simulink model "current"  (R2021a)
settings: Solver=VariableStepAuto  StartTime=0.0  StopTime=1  RelTol=1e-3
model workspace (MAT data in the model file):
  Vdc = 30
undefined symbols (not defined in the file or in its folder): f_pwm
libraries: pid_lib x5, spsControlledVoltageSourceLib x2, spsGroundLib x2, spsPermanentMagnetSynchronousMachineLib x2, spsThreePhaseVIMeasurementLib x2, spsUniversalBridgeLib x2, spsTriangleGeneratorLib x2, spsabctodq0Lib x1, spspowerguiLib x1
settings Model: SimulationMode=accelerator  Creator=Zzx  LastModifiedBy=Zzx
settings SolverCC: ZeroCrossAlgorithm=Adaptive
settings DebuggingCC: IgnoredZcDiagnostic=none

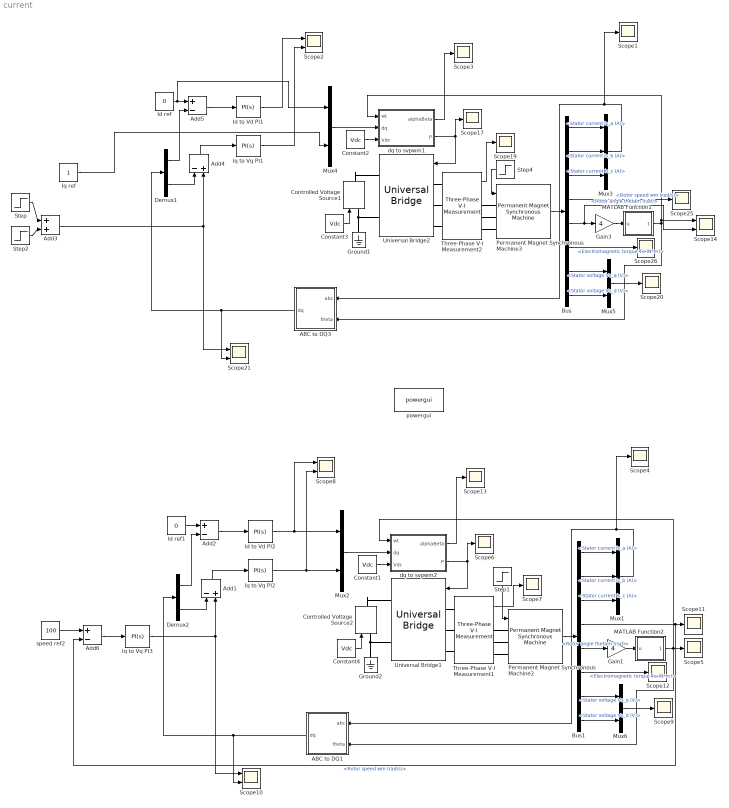
== system current ==
  ABC to DQ1 : Subsystem
  ABC to DQ3 : Subsystem
  Add1 : Sum  Inputs=-+
  Add2 : Sum  Inputs=+-
  Add3 : Sum
  Add4 : Sum  Inputs=-+
  Add5 : Sum  Inputs=+-
  Add6 : Sum  Inputs=+-
  Bus : BusSelector  OutputSignals=Stator current is_a (A),Stator current is_b (A),Stator current is_c (A),Rotor speed wm (rad/s),Rotor angle thetam (rad),Electromagnetic torque Te (N*m),Stator voltage Vs_q (V),Stator voltage Vs_d (V)
  Bus1 : BusSelector  OutputSignals=Stator current is_a (A),Stator current is_b (A),Stator current is_c (A),Rotor speed wm (rad/s),Rotor angle thetam (rad),Electromagnetic torque Te (N*m),Stator voltage Vs_q (V),Stator voltage Vs_d (V)
  Constant{1..4} (4 alike) : Constant  Value=Vdc
  Controlled Voltage Source1 : spsControlledVoltageSourceLib/Controlled Voltage Source  Initialize=on  Source_Type=DC  Amplitude=0  Phase=0  Frequency=0  Measurements=Voltage
  Controlled Voltage Source2 : spsControlledVoltageSourceLib/Controlled Voltage Source  Initialize=on  Source_Type=DC  Amplitude=0  Phase=0  Frequency=0  Measurements=Voltage
  Demux1 : Demux  Outputs=2
  Demux2 : Demux  Outputs=2
  Gain1 : Gain  Gain=4
  Gain3 : Gain  Gain=4
  Ground1 : spsGroundLib/Ground  LConnTagsString=a
  Ground2 : spsGroundLib/Ground  LConnTagsString=a
  Id ref : Constant  Value=0
  Id ref1 : Constant  Value=0
  Id to Vd PI1 : pid_lib/PID Controller  Controller=PI  Form=Parallel  TimeDomain=Continuous-time  UseExternalTs=off  SampleTime=1/f_pwm  IntegratorMethod=Forward Euler  FilterMethod=Forward Euler  ControllerParametersSource=internal  P=10  I=0  D=0  UseFilter=on  N=100  TunerSelectOption=Transfer Function Based (PID Tuner App)  InitialConditionSource=internal  InitialConditionForIntegrator=0  InitialConditionForFilter=0  DifferentiatorICPrevScaledInput=0  ExternalReset=none  TrackingMode=off  Kt=1  LimitOutput=off  SatLimitsSource=internal  UpperSaturationLimit=inf  LowerSaturationLimit=-inf  LinearizeAsGain=on  AntiWindupMode=none  Kb=1  POutMin=[]  POutMax=[]  IOutMin=[]  IOutMax=[]  DOutMin=[]  DOutMax=[]  NOutMin=[]  NOutMax=[]  SumOutMin=[]  SumOutMax=[]  SaturationOutMin=[]  SaturationOutMax=[]  PParamMin=[]  PParamMax=[]  IParamMin=[]  IParamMax=[]  DParamMin=[]  DParamMax=[]  NParamMin=[]  NParamMax=[]  KbParamMin=[]  KbParamMax=[]  KtParamMin=[]  KtParamMax=[]  KbOutMin=[]  KbOutMax=[]  KtOutMin=[]  KtOutMax=[]  IntegratorOutMin=[]  IntegratorOutMax=[]  FilterOutMin=[]  FilterOutMax=[]  SumI1OutMin=[]  SumI1OutMax=[]  SumI2OutMin=[]  SumI2OutMax=[]  SumI3OutMin=[]  SumI3OutMax=[]  SumI4OutMin=[]  SumI4OutMax=[]  SumDOutMin=[]  SumDOutMax=[]  DifferentiatorOutMin=[]  DifferentiatorOutMax=[]  FilterDiffOutCoefMin=[]  FilterDiffOutCoefMax=[]  ReciprocalOutMin=[]  ReciprocalOutMax=[]  SumDenOutMin=[]  SumDenOutMax=[]  SumNumOutMin=[]  SumNumOutMax=[]  DivideOutMin=[]  DivideOutMax=[]  UdiffTsProdOutMin=[]  UdiffTsProdOutMax=[]  NTsProdOutMin=[]  NTsProdOutMax=[]  UintegralTsProdOutMin=[]  UintegralTsProdOutMax=[]  UngainTsProdOutMin=[]  UngainTsProdOutMax=[]  IntegratorContinuousStateAttributes=''  IntegratorStateMustResolveToSignalObject=off  IntegratorRTWStateStorageClass=Auto  FilterContinuousStateAttributes=''  FilterStateMustResolveToSignalObject=off  FilterRTWStateStorageClass=Auto  ParallelPVariant=InternalParameters  IdealPVariant=Disabled  IVariant=InternalParameters  DVariant=Disabled  IntegratorVariant=Continuous  SatVariant=Disabled  AWVariant=Passthrough  PCopyVariant=Disabled  TRVariant=Disabled  FdbkBlocksVariant=Forward  IdealPFdbkVariant=Disabled  SatFdbkVariant=Disabled  DerivativeFilterVariant=Disabled  NVariant=Disabled  NCopyVariant=Disabled_SignalSpec  FilterICVariant=Disabled  IntegratorICVariant=InternalICs  ExternalResetVariant=Disabled  TRSumVariant=Passthrough  SumFdbkVariant=Disabled  SumVariant=Sum_PI  TsampFilterVariant=InternalTs  TsampNgainVariant=Passthrough  TsampIntegralVariant=Passthrough  ExternalSaturationOutDataTypeStr=Inherit: Same as second input
  Id to Vd PI2 : pid_lib/PID Controller  Controller=PI  Form=Parallel  TimeDomain=Continuous-time  UseExternalTs=off  SampleTime=1/f_pwm  IntegratorMethod=Forward Euler  FilterMethod=Forward Euler  ControllerParametersSource=internal  P=10  I=0  D=0  UseFilter=on  N=100  TunerSelectOption=Transfer Function Based (PID Tuner App)  InitialConditionSource=internal  InitialConditionForIntegrator=0  InitialConditionForFilter=0  DifferentiatorICPrevScaledInput=0  ExternalReset=none  TrackingMode=off  Kt=1  LimitOutput=off  SatLimitsSource=internal  UpperSaturationLimit=inf  LowerSaturationLimit=-inf  LinearizeAsGain=on  AntiWindupMode=none  Kb=1  POutMin=[]  POutMax=[]  IOutMin=[]  IOutMax=[]  DOutMin=[]  DOutMax=[]  NOutMin=[]  NOutMax=[]  SumOutMin=[]  SumOutMax=[]  SaturationOutMin=[]  SaturationOutMax=[]  PParamMin=[]  PParamMax=[]  IParamMin=[]  IParamMax=[]  DParamMin=[]  DParamMax=[]  NParamMin=[]  NParamMax=[]  KbParamMin=[]  KbParamMax=[]  KtParamMin=[]  KtParamMax=[]  KbOutMin=[]  KbOutMax=[]  KtOutMin=[]  KtOutMax=[]  IntegratorOutMin=[]  IntegratorOutMax=[]  FilterOutMin=[]  FilterOutMax=[]  SumI1OutMin=[]  SumI1OutMax=[]  SumI2OutMin=[]  SumI2OutMax=[]  SumI3OutMin=[]  SumI3OutMax=[]  SumI4OutMin=[]  SumI4OutMax=[]  SumDOutMin=[]  SumDOutMax=[]  DifferentiatorOutMin=[]  DifferentiatorOutMax=[]  FilterDiffOutCoefMin=[]  FilterDiffOutCoefMax=[]  ReciprocalOutMin=[]  ReciprocalOutMax=[]  SumDenOutMin=[]  SumDenOutMax=[]  SumNumOutMin=[]  SumNumOutMax=[]  DivideOutMin=[]  DivideOutMax=[]  UdiffTsProdOutMin=[]  UdiffTsProdOutMax=[]  NTsProdOutMin=[]  NTsProdOutMax=[]  UintegralTsProdOutMin=[]  UintegralTsProdOutMax=[]  UngainTsProdOutMin=[]  UngainTsProdOutMax=[]  IntegratorContinuousStateAttributes=''  IntegratorStateMustResolveToSignalObject=off  IntegratorRTWStateStorageClass=Auto  FilterContinuousStateAttributes=''  FilterStateMustResolveToSignalObject=off  FilterRTWStateStorageClass=Auto  ParallelPVariant=InternalParameters  IdealPVariant=Disabled  IVariant=InternalParameters  DVariant=Disabled  IntegratorVariant=Continuous  SatVariant=Disabled  AWVariant=Passthrough  PCopyVariant=Disabled  TRVariant=Disabled  FdbkBlocksVariant=Forward  IdealPFdbkVariant=Disabled  SatFdbkVariant=Disabled  DerivativeFilterVariant=Disabled  NVariant=Disabled  NCopyVariant=Disabled_SignalSpec  FilterICVariant=Disabled  IntegratorICVariant=InternalICs  ExternalResetVariant=Disabled  TRSumVariant=Passthrough  SumFdbkVariant=Disabled  SumVariant=Sum_PI  TsampFilterVariant=InternalTs  TsampNgainVariant=Passthrough  TsampIntegralVariant=Passthrough  ExternalSaturationOutDataTypeStr=Inherit: Same as second input
  Iq ref : Constant
  Iq to Vq PI1 : pid_lib/PID Controller  Controller=PI  Form=Parallel  TimeDomain=Continuous-time  UseExternalTs=off  SampleTime=1/f_pwm  IntegratorMethod=Forward Euler  FilterMethod=Forward Euler  ControllerParametersSource=internal  P=10  I=0  D=0  UseFilter=on  N=100  TunerSelectOption=Transfer Function Based (PID Tuner App)  InitialConditionSource=internal  InitialConditionForIntegrator=0  InitialConditionForFilter=0  DifferentiatorICPrevScaledInput=0  ExternalReset=none  TrackingMode=off  Kt=1  LimitOutput=off  SatLimitsSource=internal  UpperSaturationLimit=inf  LowerSaturationLimit=-inf  LinearizeAsGain=on  AntiWindupMode=none  Kb=1  POutMin=[]  POutMax=[]  IOutMin=[]  IOutMax=[]  DOutMin=[]  DOutMax=[]  NOutMin=[]  NOutMax=[]  SumOutMin=[]  SumOutMax=[]  SaturationOutMin=[]  SaturationOutMax=[]  PParamMin=[]  PParamMax=[]  IParamMin=[]  IParamMax=[]  DParamMin=[]  DParamMax=[]  NParamMin=[]  NParamMax=[]  KbParamMin=[]  KbParamMax=[]  KtParamMin=[]  KtParamMax=[]  KbOutMin=[]  KbOutMax=[]  KtOutMin=[]  KtOutMax=[]  IntegratorOutMin=[]  IntegratorOutMax=[]  FilterOutMin=[]  FilterOutMax=[]  SumI1OutMin=[]  SumI1OutMax=[]  SumI2OutMin=[]  SumI2OutMax=[]  SumI3OutMin=[]  SumI3OutMax=[]  SumI4OutMin=[]  SumI4OutMax=[]  SumDOutMin=[]  SumDOutMax=[]  DifferentiatorOutMin=[]  DifferentiatorOutMax=[]  FilterDiffOutCoefMin=[]  FilterDiffOutCoefMax=[]  ReciprocalOutMin=[]  ReciprocalOutMax=[]  SumDenOutMin=[]  SumDenOutMax=[]  SumNumOutMin=[]  SumNumOutMax=[]  DivideOutMin=[]  DivideOutMax=[]  UdiffTsProdOutMin=[]  UdiffTsProdOutMax=[]  NTsProdOutMin=[]  NTsProdOutMax=[]  UintegralTsProdOutMin=[]  UintegralTsProdOutMax=[]  UngainTsProdOutMin=[]  UngainTsProdOutMax=[]  IntegratorContinuousStateAttributes=''  IntegratorStateMustResolveToSignalObject=off  IntegratorRTWStateStorageClass=Auto  FilterContinuousStateAttributes=''  FilterStateMustResolveToSignalObject=off  FilterRTWStateStorageClass=Auto  ParallelPVariant=InternalParameters  IdealPVariant=Disabled  IVariant=InternalParameters  DVariant=Disabled  IntegratorVariant=Continuous  SatVariant=Disabled  AWVariant=Passthrough  PCopyVariant=Disabled  TRVariant=Disabled  FdbkBlocksVariant=Forward  IdealPFdbkVariant=Disabled  SatFdbkVariant=Disabled  DerivativeFilterVariant=Disabled  NVariant=Disabled  NCopyVariant=Disabled_SignalSpec  FilterICVariant=Disabled  IntegratorICVariant=InternalICs  ExternalResetVariant=Disabled  TRSumVariant=Passthrough  SumFdbkVariant=Disabled  SumVariant=Sum_PI  TsampFilterVariant=InternalTs  TsampNgainVariant=Passthrough  TsampIntegralVariant=Passthrough  ExternalSaturationOutDataTypeStr=Inherit: Same as second input
  Iq to Vq PI2 : pid_lib/PID Controller  Controller=PI  Form=Parallel  TimeDomain=Continuous-time  UseExternalTs=off  SampleTime=1/f_pwm  IntegratorMethod=Forward Euler  FilterMethod=Forward Euler  ControllerParametersSource=internal  P=10  I=0  D=0  UseFilter=on  N=100  TunerSelectOption=Transfer Function Based (PID Tuner App)  InitialConditionSource=internal  InitialConditionForIntegrator=0  InitialConditionForFilter=0  DifferentiatorICPrevScaledInput=0  ExternalReset=none  TrackingMode=off  Kt=1  LimitOutput=off  SatLimitsSource=internal  UpperSaturationLimit=inf  LowerSaturationLimit=-inf  LinearizeAsGain=on  AntiWindupMode=none  Kb=1  POutMin=[]  POutMax=[]  IOutMin=[]  IOutMax=[]  DOutMin=[]  DOutMax=[]  NOutMin=[]  NOutMax=[]  SumOutMin=[]  SumOutMax=[]  SaturationOutMin=[]  SaturationOutMax=[]  PParamMin=[]  PParamMax=[]  IParamMin=[]  IParamMax=[]  DParamMin=[]  DParamMax=[]  NParamMin=[]  NParamMax=[]  KbParamMin=[]  KbParamMax=[]  KtParamMin=[]  KtParamMax=[]  KbOutMin=[]  KbOutMax=[]  KtOutMin=[]  KtOutMax=[]  IntegratorOutMin=[]  IntegratorOutMax=[]  FilterOutMin=[]  FilterOutMax=[]  SumI1OutMin=[]  SumI1OutMax=[]  SumI2OutMin=[]  SumI2OutMax=[]  SumI3OutMin=[]  SumI3OutMax=[]  SumI4OutMin=[]  SumI4OutMax=[]  SumDOutMin=[]  SumDOutMax=[]  DifferentiatorOutMin=[]  DifferentiatorOutMax=[]  FilterDiffOutCoefMin=[]  FilterDiffOutCoefMax=[]  ReciprocalOutMin=[]  ReciprocalOutMax=[]  SumDenOutMin=[]  SumDenOutMax=[]  SumNumOutMin=[]  SumNumOutMax=[]  DivideOutMin=[]  DivideOutMax=[]  UdiffTsProdOutMin=[]  UdiffTsProdOutMax=[]  NTsProdOutMin=[]  NTsProdOutMax=[]  UintegralTsProdOutMin=[]  UintegralTsProdOutMax=[]  UngainTsProdOutMin=[]  UngainTsProdOutMax=[]  IntegratorContinuousStateAttributes=''  IntegratorStateMustResolveToSignalObject=off  IntegratorRTWStateStorageClass=Auto  FilterContinuousStateAttributes=''  FilterStateMustResolveToSignalObject=off  FilterRTWStateStorageClass=Auto  ParallelPVariant=InternalParameters  IdealPVariant=Disabled  IVariant=InternalParameters  DVariant=Disabled  IntegratorVariant=Continuous  SatVariant=Disabled  AWVariant=Passthrough  PCopyVariant=Disabled  TRVariant=Disabled  FdbkBlocksVariant=Forward  IdealPFdbkVariant=Disabled  SatFdbkVariant=Disabled  DerivativeFilterVariant=Disabled  NVariant=Disabled  NCopyVariant=Disabled_SignalSpec  FilterICVariant=Disabled  IntegratorICVariant=InternalICs  ExternalResetVariant=Disabled  TRSumVariant=Passthrough  SumFdbkVariant=Disabled  SumVariant=Sum_PI  TsampFilterVariant=InternalTs  TsampNgainVariant=Passthrough  TsampIntegralVariant=Passthrough  ExternalSaturationOutDataTypeStr=Inherit: Same as second input
  Iq to Vq PI3 : pid_lib/PID Controller  Controller=PI  Form=Parallel  TimeDomain=Continuous-time  UseExternalTs=off  SampleTime=1/f_pwm  IntegratorMethod=Forward Euler  FilterMethod=Forward Euler  ControllerParametersSource=internal  P=10  I=0  D=0  UseFilter=on  N=100  TunerSelectOption=Transfer Function Based (PID Tuner App)  InitialConditionSource=internal  InitialConditionForIntegrator=0  InitialConditionForFilter=0  DifferentiatorICPrevScaledInput=0  ExternalReset=none  TrackingMode=off  Kt=1  LimitOutput=off  SatLimitsSource=internal  UpperSaturationLimit=inf  LowerSaturationLimit=-inf  LinearizeAsGain=on  AntiWindupMode=none  Kb=1  POutMin=[]  POutMax=[]  IOutMin=[]  IOutMax=[]  DOutMin=[]  DOutMax=[]  NOutMin=[]  NOutMax=[]  SumOutMin=[]  SumOutMax=[]  SaturationOutMin=[]  SaturationOutMax=[]  PParamMin=[]  PParamMax=[]  IParamMin=[]  IParamMax=[]  DParamMin=[]  DParamMax=[]  NParamMin=[]  NParamMax=[]  KbParamMin=[]  KbParamMax=[]  KtParamMin=[]  KtParamMax=[]  KbOutMin=[]  KbOutMax=[]  KtOutMin=[]  KtOutMax=[]  IntegratorOutMin=[]  IntegratorOutMax=[]  FilterOutMin=[]  FilterOutMax=[]  SumI1OutMin=[]  SumI1OutMax=[]  SumI2OutMin=[]  SumI2OutMax=[]  SumI3OutMin=[]  SumI3OutMax=[]  SumI4OutMin=[]  SumI4OutMax=[]  SumDOutMin=[]  SumDOutMax=[]  DifferentiatorOutMin=[]  DifferentiatorOutMax=[]  FilterDiffOutCoefMin=[]  FilterDiffOutCoefMax=[]  ReciprocalOutMin=[]  ReciprocalOutMax=[]  SumDenOutMin=[]  SumDenOutMax=[]  SumNumOutMin=[]  SumNumOutMax=[]  DivideOutMin=[]  DivideOutMax=[]  UdiffTsProdOutMin=[]  UdiffTsProdOutMax=[]  NTsProdOutMin=[]  NTsProdOutMax=[]  UintegralTsProdOutMin=[]  UintegralTsProdOutMax=[]  UngainTsProdOutMin=[]  UngainTsProdOutMax=[]  IntegratorContinuousStateAttributes=''  IntegratorStateMustResolveToSignalObject=off  IntegratorRTWStateStorageClass=Auto  FilterContinuousStateAttributes=''  FilterStateMustResolveToSignalObject=off  FilterRTWStateStorageClass=Auto  ParallelPVariant=InternalParameters  IdealPVariant=Disabled  IVariant=InternalParameters  DVariant=Disabled  IntegratorVariant=Continuous  SatVariant=Disabled  AWVariant=Passthrough  PCopyVariant=Disabled  TRVariant=Disabled  FdbkBlocksVariant=Forward  IdealPFdbkVariant=Disabled  SatFdbkVariant=Disabled  DerivativeFilterVariant=Disabled  NVariant=Disabled  NCopyVariant=Disabled_SignalSpec  FilterICVariant=Disabled  IntegratorICVariant=InternalICs  ExternalResetVariant=Disabled  TRSumVariant=Passthrough  SumFdbkVariant=Disabled  SumVariant=Sum_PI  TsampFilterVariant=InternalTs  TsampNgainVariant=Passthrough  TsampIntegralVariant=Passthrough  ExternalSaturationOutDataTypeStr=Inherit: Same as second input
  MATLAB Function1 : MATLAB Function  TreatAsAtomicUnit=on
  MATLAB Function2 : MATLAB Function  TreatAsAtomicUnit=on
  Mux1 : Mux  Inputs=3
  Mux{2,4..6} (4 alike) : Mux  Inputs=2
  Mux3 : Mux  Inputs=3
  Permanent Magnet Synchronous Machine2 : spsPermanentMagnetSynchronousMachineLib/Permanent Magnet Synchronous Machine  NbPhases=3  FluxDistribution=Sinusoidal  RotorType=Round  MechanicalLoad=Torque Tm  PresetModel=No  ShowDetailedParameters=on  MeasurementBus=off  Resistance=0.89  Inductance=8.5e-3  dqInductances=[8.5e-3,8.5e-3]  La=0.00062  MachineConstant=Voltage Constant (V_peak L-L / krpm)  Flux=0.0056925  VoltageCst=4.13  TorqueCst=0.034155  Flat=120  Mechanical=[ 0.8e-3, 0 4]  PolePairs=4  InitialConditions=[0,0, 0,0]  InitialConditions5ph=[0 0 0 0 0 0]  RefAngle=Aligned with phase A axis (original Park)  IterativeDiscreteModel=Trapezoidal non iterative  TsBlock=-1  TsPowergui=0
  Permanent Magnet Synchronous Machine3 : spsPermanentMagnetSynchronousMachineLib/Permanent Magnet Synchronous Machine  NbPhases=3  FluxDistribution=Sinusoidal  RotorType=Round  MechanicalLoad=Torque Tm  PresetModel=No  ShowDetailedParameters=on  MeasurementBus=off  Resistance=0.89  Inductance=8.5e-3  dqInductances=[8.5e-3,8.5e-3]  La=0.00062  MachineConstant=Voltage Constant (V_peak L-L / krpm)  Flux=0.0056925  VoltageCst=4.13  TorqueCst=0.034155  Flat=120  Mechanical=[ 0.8e-3, 0 4]  PolePairs=4  InitialConditions=[0,0, 0,0]  InitialConditions5ph=[0 0 0 0 0 0]  RefAngle=Aligned with phase A axis (original Park)  IterativeDiscreteModel=Trapezoidal non iterative  TsBlock=-1  TsPowergui=0
  Scope{1,3..7,9,11..13,17,19..20,25..26} (15 alike) : Scope
  Scope{2,8,10,14,21} (5 alike) : Scope  NumInputPorts=2
  Step : Step  Time=0.25  Before=0.5  After=2  SampleTime=0
  Step1 : Step  Time=0.5  After=0  SampleTime=0
  Step2 : Step  Time=0.75  After=-1  SampleTime=0
  Step4 : Step  Time=0.5  After=0  SampleTime=0
  Three-Phase V-I Measurement1 : spsThreePhaseVIMeasurementLib/Three-Phase V-I Measurement  VoltageMeasurement=phase-to-ground  SetLabelV=off  LabelV=Vabc  Vpu=off  VpuLL=off  CurrentMeasurement=yes  SetLabelI=off  LabelI=Iabc  Ipu=off  Pbase=100e6  Vbase=500e3  OutputType=Complex  PhasorSimulation=off  PSBequivalent=0
  Three-Phase V-I Measurement2 : spsThreePhaseVIMeasurementLib/Three-Phase V-I Measurement  VoltageMeasurement=phase-to-ground  SetLabelV=off  LabelV=Vabc  Vpu=off  VpuLL=off  CurrentMeasurement=yes  SetLabelI=off  LabelI=Iabc  Ipu=off  Pbase=100e6  Vbase=500e3  OutputType=Complex  PhasorSimulation=off  PSBequivalent=0
  Universal Bridge1 : spsUniversalBridgeLib/Universal Bridge  Arms=3  SnubberResistance=1e5  SnubberCapacitance=inf  Device=IGBT / Diodes  Ron=1e-3  Lon=0  ForwardVoltages="[  0  0  ]"  ForwardVoltage=0  GTOparameters=[ 10e-6 , 20e-6 ]  IGBTparameters=[ 1e-6 , 2e-6 ]  Measurements=None  Measurements_2=None  converterType=Rectifier
  Universal Bridge2 : spsUniversalBridgeLib/Universal Bridge  Arms=3  SnubberResistance=1e5  SnubberCapacitance=inf  Device=IGBT / Diodes  Ron=1e-3  Lon=0  ForwardVoltages="[  0  0  ]"  ForwardVoltage=0  GTOparameters=[ 10e-6 , 20e-6 ]  IGBTparameters=[ 1e-6 , 2e-6 ]  Measurements=None  Measurements_2=None  converterType=Rectifier
  dq to svpwm1 : Subsystem
  dq to svpwm2 : Subsystem
  powergui : spspowerguiLib/powergui  Priority=1  SimulationMode=Continuous  SampleTime=50e-6  frequency=60  Iterations=50  frequencyindice=0  Pbase=100e6  ErrMax=1e-4  UnitsV=kV  UnitsW=MW  buscounter=0  FunctionMessages=off  echomessages=off  EnableUseOfTLC=off  CurrentSourceSwitches=off  DisableSnubberDevices=off  DisableRonSwitches=off  DisableVfSwitches=off  DisplayEquations=off  AutomaticDiscreteSolvers=off  SolverType=Tustin/Backward Euler (TBE)  Interpol=off  ExternalGateDelay=off  methode=off  Ts=100  x0status=blocks  SPID=on  SwTol=0  HookPort=off  NonlinearTolerance=1e-4  nMaxIteration=100  ContinueOnMaxIteration=off  RestoreLinks=warning  ResistiveCurrentMeasurement=off  Frange=[0:2:500]  Ylog=off  Xlog=on  ShowGrid=off  save=off  variable=ZData  structure=0  ZoomFFT=off  StartTime=0.0  cycles=1  DisplayStyle=1  fundamental=60  FreqAxis=off  MaxFrequency=1000  frequencyindicesteady=1  RmsSteady=1  display=off
  speed ref2 : Constant  Value=100
  wires:
  Three-Phase V-I Measurement2/1 -> Scope19/1
  Id to Vd PI1/1 -> Scope2/1
  Iq to Vq PI1/1 -> Scope2/2
  Step4/1 -> Permanent Magnet Synchronous Machine3/1
  Bus/7 -> Mux5/1  "<Stator voltage Vs_q (V)>"
  Bus/2 -> Mux3/2  "<Stator current is_b (A)>"
  Bus/5 -> Scope14/2, Gain3/1  "<Rotor angle thetam (rad)>"
  Bus/6 -> Scope26/1  "<Electromagnetic torque Te (N*m)>"
  Mux4/1 -> dq to svpwm1/2(dq)
  ABC to DQ3/1(dq) -> Scope21/2, Demux1/1
  Constant2/1 -> dq to svpwm1/3(Vdc)
  Bus/8 -> Mux5/2  "<Stator voltage Vs_d (V)>"
  Mux3/1 -> ABC to DQ3/1(abc), Scope1/1
  Gain3/1 -> MATLAB Function1/1(u)
  Bus/1 -> Mux3/1  "<Stator current is_a (A)>"
  Mux5/1 -> Scope20/1
  Add4/1 -> Iq to Vq PI1/1
  Bus/4 -> Scope25/1  "<Rotor speed wm (rad/s)>"
  Bus/3 -> Mux3/3  "<Stator current is_c (A)>"
  Demux1/2 -> Add4/1
  Id ref/1 -> Mux4/1, Add5/1
  MATLAB Function1/1(theta) -> Scope14/1, dq to svpwm1/1(wt), ABC to DQ3/2(theta)
  Add5/1 -> Id to Vd PI1/1
  Demux1/1 -> Add5/2
  Constant3/1 -> Controlled Voltage Source1/1
  dq to svpwm1/2(P) -> Scope17/1, Universal Bridge2/1
  Permanent Magnet Synchronous Machine3/1 -> Bus/1
  dq to svpwm1/1(alphaBeta) -> Scope3/1
  Add3/1 -> Scope21/1, Add4/2
  Step/1 -> Add3/1
  Step2/1 -> Add3/2
  Step1/1 -> Permanent Magnet Synchronous Machine2/1
  Permanent Magnet Synchronous Machine2/1 -> Bus1/1
  dq to svpwm2/2(P) -> Scope6/1, Universal Bridge1/1
  Demux2/1 -> Add2/2
  Id ref1/1 -> Add2/1
  Demux2/2 -> Add1/1
  Gain1/1 -> MATLAB Function2/1(u)
  Mux6/1 -> Scope9/1
  Bus1/3 -> Mux1/3  "<Stator current is_c (A)>"
  MATLAB Function2/1(theta) -> dq to svpwm2/1(wt), ABC to DQ1/2(theta), Scope5/1
  Bus1/1 -> Mux1/1  "<Stator current is_a (A)>"
  Bus1/8 -> Mux6/2  "<Stator voltage Vs_d (V)>"
  Bus1/5 -> Gain1/1  "<Rotor angle thetam (rad)>"
  Constant1/1 -> dq to svpwm2/3(Vdc)
  Add1/1 -> Iq to Vq PI2/1
  Constant4/1 -> Controlled Voltage Source2/1
  ABC to DQ1/1(dq) -> Scope10/2, Demux2/1
  Mux2/1 -> dq to svpwm2/2(dq)
  Bus1/6 -> Scope12/1  "<Electromagnetic torque Te (N*m)>"
  Three-Phase V-I Measurement1/1 -> Scope7/1
  Id to Vd PI2/1 -> Mux2/1, Scope8/1
  Iq to Vq PI2/1 -> Mux2/2, Scope8/2
  Bus1/2 -> Mux1/2  "<Stator current is_b (A)>"
  Mux1/1 -> ABC to DQ1/1(abc), Scope4/1
  Bus1/7 -> Mux6/1  "<Stator voltage Vs_q (V)>"
  dq to svpwm2/1(alphaBeta) -> Scope13/1
  Add2/1 -> Id to Vd PI2/1
  Bus1/4 -> Add6/2, Scope11/1  "<Rotor speed wm (rad/s)>"
  Iq to Vq PI3/1 -> Add1/2, Scope10/1
  speed ref2/1 -> Add6/1
  Add6/1 -> Iq to Vq PI3/1
  Iq ref/1 -> Mux4/2
  connections:
  Controlled Voltage Source1/LConn1 -- Ground1/LConn1 -- Universal Bridge2/RConn2
  Three-Phase V-I Measurement2/LConn1 -- Universal Bridge2/LConn1
  Permanent Magnet Synchronous Machine3/LConn3 -- Three-Phase V-I Measurement2/RConn3
  Three-Phase V-I Measurement2/LConn2 -- Universal Bridge2/LConn2
  Controlled Voltage Source1/RConn1 -- Universal Bridge2/RConn1
  Permanent Magnet Synchronous Machine3/LConn2 -- Three-Phase V-I Measurement2/RConn2
  Three-Phase V-I Measurement2/LConn3 -- Universal Bridge2/LConn3
  Permanent Magnet Synchronous Machine3/LConn1 -- Three-Phase V-I Measurement2/RConn1
  Controlled Voltage Source2/LConn1 -- Ground2/LConn1 -- Universal Bridge1/RConn2
  Permanent Magnet Synchronous Machine2/LConn2 -- Three-Phase V-I Measurement1/RConn2
  Permanent Magnet Synchronous Machine2/LConn1 -- Three-Phase V-I Measurement1/RConn1
  Controlled Voltage Source2/RConn1 -- Universal Bridge1/RConn1
  Three-Phase V-I Measurement1/LConn1 -- Universal Bridge1/LConn1
  Three-Phase V-I Measurement1/LConn2 -- Universal Bridge1/LConn2
  Three-Phase V-I Measurement1/LConn3 -- Universal Bridge1/LConn3
  Permanent Magnet Synchronous Machine2/LConn3 -- Three-Phase V-I Measurement1/RConn3

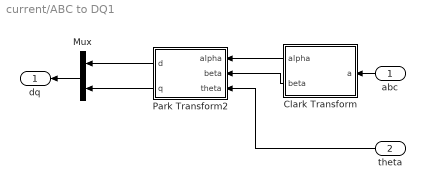
== system current/ABC to DQ1 ==
  abc : Inport
  theta : Inport  Port=2
  Clark Transform : MATLAB Function  TreatAsAtomicUnit=on
  Mux : Mux  Inputs=2
  Park Transform2 : MATLAB Function  TreatAsAtomicUnit=on
  dq : Outport
  wires:
  Clark Transform/1(alpha) -> Park Transform2/1(alpha)
  Clark Transform/2(beta) -> Park Transform2/2(beta)
  abc/1 -> Clark Transform/1(a)
  theta/1 -> Park Transform2/3(theta)
  Park Transform2/1(d) -> Mux/1
  Park Transform2/2(q) -> Mux/2
  Mux/1 -> dq/1

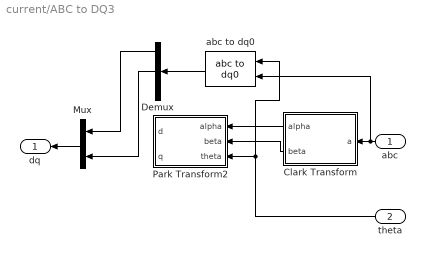
== system current/ABC to DQ3 ==
  abc : Inport
  theta : Inport  Port=2
  Clark Transform : MATLAB Function  TreatAsAtomicUnit=on
  Demux : Demux  Outputs=3
  Mux : Mux  Inputs=2
  Park Transform2 : MATLAB Function  TreatAsAtomicUnit=on
  abc to dq0 : spsabctodq0Lib/abc to dq0  Alignment=90 degrees behind phase A axis
  dq : Outport
  wires:
  Clark Transform/1(alpha) -> Park Transform2/1(alpha)
  Clark Transform/2(beta) -> Park Transform2/2(beta)
  abc/1 -> abc to dq0/1, Clark Transform/1(a)
  theta/1 -> abc to dq0/2, Park Transform2/3(theta)
  Mux/1 -> dq/1
  abc to dq0/1 -> Demux/1
  Demux/1 -> Mux/1
  Demux/2 -> Mux/2

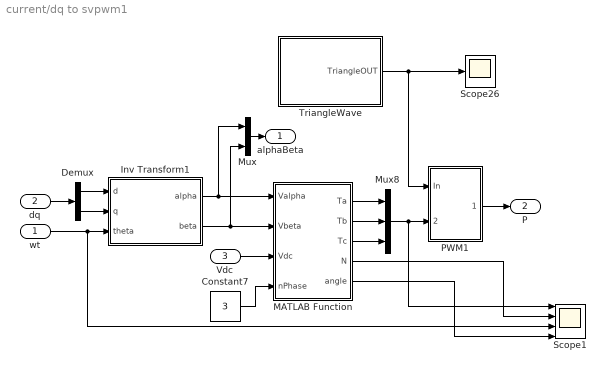
== system current/dq to svpwm1 ==
  wt : Inport
  dq : Inport  Port=2
  Vdc : Inport  Port=3
  Constant7 : Constant  Value=3
  Demux : Demux  Outputs=2
  Inv Transform1 : MATLAB Function  TreatAsAtomicUnit=on
  MATLAB Function : MATLAB Function  TreatAsAtomicUnit=on
  Mux : Mux  Inputs=2
  Mux8 : Mux  Inputs=3
  PWM1 : Subsystem
  Scope1 : Scope  NumInputPorts=4
  Scope26 : Scope
  TriangleWave : Subsystem
  alphaBeta : Outport
  P : Outport  Port=2
  wires:
  Inv Transform1/2(beta) -> MATLAB Function/2(Vbeta), Mux/2
  wt/1 -> Scope1/3, Inv Transform1/3(theta)
  dq/1 -> Demux/1
  Inv Transform1/1(alpha) -> MATLAB Function/1(Valpha), Mux/1
  MATLAB Function/1(Ta) -> Mux8/1
  MATLAB Function/3(Tc) -> Mux8/3
  MATLAB Function/2(Tb) -> Mux8/2
  Vdc/1 -> MATLAB Function/3(Vdc)
  Constant7/1 -> MATLAB Function/4(nPhase)
  PWM1/1(PWM) -> P/1
  Mux8/1 -> PWM1/2(Tcm123), Scope1/1
  Demux/1 -> Inv Transform1/1(d)
  Demux/2 -> Inv Transform1/2(q)
  Mux/1 -> alphaBeta/1
  TriangleWave/1(TriangleOUT) -> Scope26/1, PWM1/1(In)
  MATLAB Function/4(N) -> Scope1/2
  MATLAB Function/5(angle) -> Scope1/4

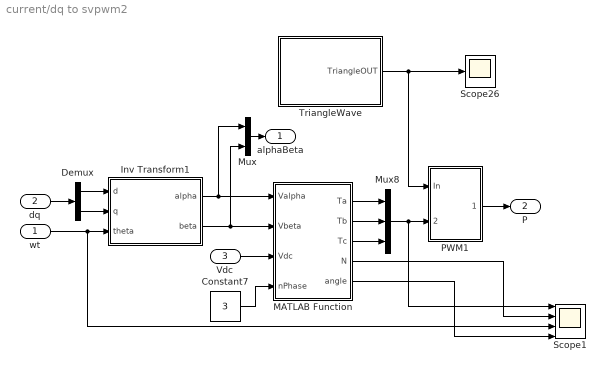
== system current/dq to svpwm2 ==
  wt : Inport
  dq : Inport  Port=2
  Vdc : Inport  Port=3
  Constant7 : Constant  Value=3
  Demux : Demux  Outputs=2
  Inv Transform1 : MATLAB Function  TreatAsAtomicUnit=on
  MATLAB Function : MATLAB Function  TreatAsAtomicUnit=on
  Mux : Mux  Inputs=2
  Mux8 : Mux  Inputs=3
  PWM1 : Subsystem
  Scope1 : Scope  NumInputPorts=4
  Scope26 : Scope
  TriangleWave : Subsystem
  alphaBeta : Outport
  P : Outport  Port=2
  wires:
  Inv Transform1/2(beta) -> MATLAB Function/2(Vbeta), Mux/2
  wt/1 -> Scope1/3, Inv Transform1/3(theta)
  dq/1 -> Demux/1
  Inv Transform1/1(alpha) -> MATLAB Function/1(Valpha), Mux/1
  MATLAB Function/1(Ta) -> Mux8/1
  MATLAB Function/3(Tc) -> Mux8/3
  MATLAB Function/2(Tb) -> Mux8/2
  Vdc/1 -> MATLAB Function/3(Vdc)
  Constant7/1 -> MATLAB Function/4(nPhase)
  PWM1/1(PWM) -> P/1
  Mux8/1 -> PWM1/2(Tcm123), Scope1/1
  Demux/1 -> Inv Transform1/1(d)
  Demux/2 -> Inv Transform1/2(q)
  Mux/1 -> alphaBeta/1
  TriangleWave/1(TriangleOUT) -> Scope26/1, PWM1/1(In)
  MATLAB Function/4(N) -> Scope1/2
  MATLAB Function/5(angle) -> Scope1/4

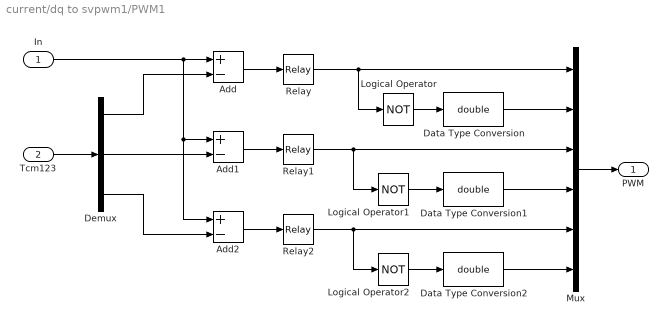
== system current/dq to svpwm1/PWM1 ==
  In : Inport
  Tcm123 : Inport  Port=2
  Add : Sum  Inputs=+-
  Add1 : Sum  Inputs=+-
  Add2 : Sum  Inputs=+-
  Data Type Conversion : DataTypeConversion  OutDataTypeStr=double
  Data Type Conversion1 : DataTypeConversion  OutDataTypeStr=double
  Data Type Conversion2 : DataTypeConversion  OutDataTypeStr=double
  Demux : Demux  Outputs=3
  Logical Operator : Logic  Operator=NOT  AllPortsSameDT=off  OutDataTypeStr=boolean
  Logical Operator1 : Logic  Operator=NOT  AllPortsSameDT=off  OutDataTypeStr=boolean
  Logical Operator2 : Logic  Operator=NOT  AllPortsSameDT=off  OutDataTypeStr=boolean
  Mux : Mux  Inputs=6
  Relay : Relay
  Relay1 : Relay
  Relay2 : Relay
  PWM : Outport
  wires:
  Demux/3 -> Add2/2
  Demux/2 -> Add1/2
  Demux/1 -> Add/2
  Relay2/1 -> Mux/5, Logical Operator2/1
  Relay1/1 -> Mux/3, Logical Operator1/1
  Relay/1 -> Logical Operator/1, Mux/1
  Mux/1 -> PWM/1
  Data Type Conversion/1 -> Mux/2
  Data Type Conversion1/1 -> Mux/4
  Data Type Conversion2/1 -> Mux/6
  Logical Operator2/1 -> Data Type Conversion2/1
  Logical Operator1/1 -> Data Type Conversion1/1
  Logical Operator/1 -> Data Type Conversion/1
  Add1/1 -> Relay1/1
  Add2/1 -> Relay2/1
  Add/1 -> Relay/1
  In/1 -> Add/1, Add2/1, Add1/1
  Tcm123/1 -> Demux/1

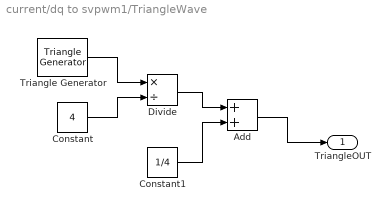
== system current/dq to svpwm1/TriangleWave ==
  Add : Sum
  Constant : Constant  Value=4
  Constant1 : Constant  Value=1/4
  Divide : Product  Inputs=*/
  Triangle Generator : spsTriangleGeneratorLib/Triangle Generator  Freq=f_pwm  Phase=0  Ts=0
  TriangleOUT : Outport
  wires:
  Add/1 -> TriangleOUT/1
  Constant/1 -> Divide/2
  Constant1/1 -> Add/2
  Divide/1 -> Add/1
  Triangle Generator/1 -> Divide/1

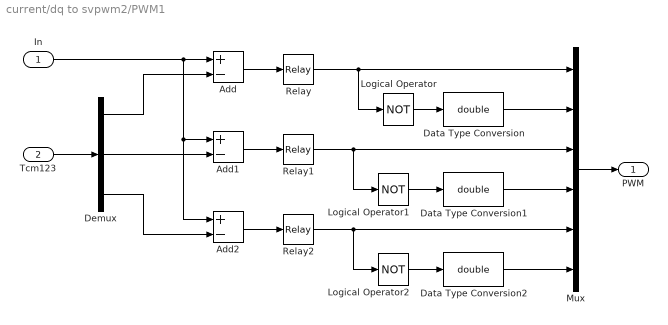
== system current/dq to svpwm2/PWM1 ==
  In : Inport
  Tcm123 : Inport  Port=2
  Add : Sum  Inputs=+-
  Add1 : Sum  Inputs=+-
  Add2 : Sum  Inputs=+-
  Data Type Conversion : DataTypeConversion  OutDataTypeStr=double
  Data Type Conversion1 : DataTypeConversion  OutDataTypeStr=double
  Data Type Conversion2 : DataTypeConversion  OutDataTypeStr=double
  Demux : Demux  Outputs=3
  Logical Operator : Logic  Operator=NOT  AllPortsSameDT=off  OutDataTypeStr=boolean
  Logical Operator1 : Logic  Operator=NOT  AllPortsSameDT=off  OutDataTypeStr=boolean
  Logical Operator2 : Logic  Operator=NOT  AllPortsSameDT=off  OutDataTypeStr=boolean
  Mux : Mux  Inputs=6
  Relay : Relay
  Relay1 : Relay
  Relay2 : Relay
  PWM : Outport
  wires:
  Demux/3 -> Add2/2
  Demux/2 -> Add1/2
  Demux/1 -> Add/2
  Relay2/1 -> Mux/5, Logical Operator2/1
  Relay1/1 -> Mux/3, Logical Operator1/1
  Relay/1 -> Logical Operator/1, Mux/1
  Mux/1 -> PWM/1
  Data Type Conversion/1 -> Mux/2
  Data Type Conversion1/1 -> Mux/4
  Data Type Conversion2/1 -> Mux/6
  Logical Operator2/1 -> Data Type Conversion2/1
  Logical Operator1/1 -> Data Type Conversion1/1
  Logical Operator/1 -> Data Type Conversion/1
  Add1/1 -> Relay1/1
  Add2/1 -> Relay2/1
  Add/1 -> Relay/1
  In/1 -> Add/1, Add2/1, Add1/1
  Tcm123/1 -> Demux/1

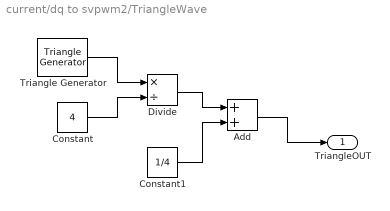
== system current/dq to svpwm2/TriangleWave ==
  Add : Sum
  Constant : Constant  Value=4
  Constant1 : Constant  Value=1/4
  Divide : Product  Inputs=*/
  Triangle Generator : spsTriangleGeneratorLib/Triangle Generator  Freq=f_pwm  Phase=0  Ts=0
  TriangleOUT : Outport
  wires:
  Add/1 -> TriangleOUT/1
  Constant/1 -> Divide/2
  Constant1/1 -> Add/2
  Divide/1 -> Add/1
  Triangle Generator/1 -> Divide/1

== matlab function current/ABC to DQ1/Clark Transform ==
  data: a input; alpha output; beta output
function [alpha,beta] = fcn(a)

alpha = a(1)-0.5*a(2)-0.5*a(3);
beta = 0.5*sqrt(3)*a(2)-0.5*sqrt(3)*a(3);

== matlab function current/ABC to DQ1/Park Transform2 ==
  data: alpha input; d output; beta input; theta input; q output
function [d,q] = fcn(alpha,beta,theta)

d = alpha*cos(theta)+beta*sin(theta);
q = -alpha*sin(theta)+beta*cos(theta);

== matlab function current/MATLAB Function2 ==
  data: u input; theta output
function theta = fcn(u)

theta = mod(u,2*pi);

== matlab function current/dq to svpwm2/Inv Transform1 ==
  data: d input; q input; alpha output; theta input; beta output
function [alpha,beta] = fcn(d,q,theta)

alpha = d*cos(theta)-q*sin(theta);
beta = d*sin(theta)+q*cos(theta);

== matlab function current/dq to svpwm2/MATLAB Function ==
  data: Valpha input; Ta output; Vbeta input; Vdc input; nPhase input; Tb output; Tc output; N output; angle output
function [Ta, Tb, Tc, N,angle ] = FindT(Valpha, Vbeta, Vdc, nPhase)
% from Valpha Vbeta calculates the 
% T0 - the idle time
% T1 - the time at Vi
% T2 - the time at V(i+1) = Vj

nPhase = floor(nPhase);
if nPhase <3
    nPhase = 3;
end

Valpha = Valpha / Vdc;
Vbeta = Vbeta/Vdc;

angle = atan2(Vbeta,Valpha);
%if Valpha<0
  %  angle = angle + pi;
%end
%angle = angle - 0.5*pi;
if angle <0
    angle = angle + 2*pi;
end

i = floor(angle/pi*nPhase);
Vi = exp(1j*pi*i/nPhase);
Vj = exp(1j*pi*(i+1)/nPhase);

Vm = (Vi+Vj)/2;
Vmabs = abs(Vm);
Vout = Valpha + 1j*Vbeta;
%Vabs = abs(Vout);

Vout_para = real(Vout * conj(Vm))/Vmabs;
if Vout_para > Vmabs
    Vout = Vout /Vout_para *Vmabs;
    Vout_para  = Vmabs;
end

T0 = 1- Vout_para / Vmabs;
Vom = Vout / Vout_para *Vmabs - Vm;
T2 = (real(Vom/(Vj-Vi))+0.5) * (1-T0);
T1 = 1-T0-T2;
N = mod(i,2*nPhase)+1;


Tall = [T0/4 T1/2+T0/4 T2/2+T0/4 T1/2+T2/2+T0/4];

switch (N)
case 1
    Ta = Tall(1);
    Tb = Tall(2);
    Tc = Tall(4);
case 2
    Ta = Tall(3);
    Tb = Tall(1);
    Tc = Tall(4);
case 3
    Ta = Tall(4);
    Tb = Tall(1);
    Tc = Tall(2);
case 4
    Ta = Tall(4);
    Tb = Tall(3);
    Tc = Tall(1);
case 5
    Ta = Tall(2);
    Tb = Tall(4);
    Tc = Tall(1);
case 6
    Ta = Tall(1);
    Tb = Tall(4);
    Tc = Tall(3);
otherwise
    Ta = 0;
    Tb = 0;
    Tc = 0;
            
end

end

== matlab function current/ABC to DQ3/Clark Transform ==
  data: a input; alpha output; beta output
function [alpha,beta] = fcn(a)

alpha = a(1)-0.5*a(2)-0.5*a(3);
beta = 0.5*sqrt(3)*a(2)-0.5*sqrt(3)*a(3);

== matlab function current/ABC to DQ3/Park Transform2 ==
  data: alpha input; d output; beta input; theta input; q output
function [d,q] = fcn(alpha,beta,theta)

d = alpha*cos(theta)+beta*sin(theta);
q = -alpha*sin(theta)+beta*cos(theta);

== matlab function current/MATLAB Function1 ==
  data: u input; theta output
function theta = fcn(u)

theta = mod(u,2*pi);

== matlab function current/dq to svpwm1/Inv Transform1 ==
  data: d input; q input; alpha output; theta input; beta output
function [alpha,beta] = fcn(d,q,theta)

alpha = d*cos(theta)-q*sin(theta);
beta = d*sin(theta)+q*cos(theta);

== matlab function current/dq to svpwm1/MATLAB Function ==
  data: Valpha input; Ta output; Vbeta input; Vdc input; nPhase input; Tb output; Tc output; N output; angle output
function [Ta, Tb, Tc, N,angle ] = FindT(Valpha, Vbeta, Vdc, nPhase)
% from Valpha Vbeta calculates the 
% T0 - the idle time
% T1 - the time at Vi
% T2 - the time at V(i+1) = Vj

nPhase = floor(nPhase);
if nPhase <3
    nPhase = 3;
end

Valpha = Valpha / Vdc;
Vbeta = Vbeta/Vdc;

angle = atan(Vbeta/Valpha);
if Valpha<0
    angle = angle + pi;
end
if angle <0
    angle = angle + 2*pi;
end

i = floor(angle/pi*nPhase);
Vi = exp(1j*pi*i/nPhase);
Vj = exp(1j*pi*(i+1)/nPhase);
%fprintf("sector %d\n", i);
%fprintf("Vi %f,%f | Vj %f, %f\n",real(Vi),imag(Vi),real(Vj),imag(Vj));

Vm = (Vi+Vj)/2;
Vmabs = abs(Vm);
Vout = Valpha + 1j*Vbeta;
%Vabs = abs(Vout);
%fprintf("Vm %f,%f Vmabs %f\n",real(Vm),imag(Vm),Vmabs);
Vout_para = real(Vout * conj(Vm))/Vmabs;
%fprintf("Vout %f,%f Vout_para %f\n",real(Vout),imag(Vout),Vout_para);
if Vout_para > Vmabs
    Vout = Vout /Vout_para *Vmabs;
    Vout_para  = Vmabs;
end
%fprintf("Vout %f,%f Vout_para %f\n",real(Vout),imag(Vout),Vout_para);

T0 = 1- Vout_para / Vmabs;
Vom = Vout / Vout_para *Vmabs - Vm;
T2 = (real(Vom/(Vj-Vi))+0.5) * (1-T0);
T1 = 1-T0-T2;
N = mod(i,2*nPhase);
%fprintf("Vom %f,%f\n",real(Vom),imag(Vom));
%fprintf("T0 %f,T2 %f,T1 %f,N %d\n",T0,T2,T1,N);

Tall = [T0/4 T1/2+T0/4 T2/2+T0/4 T1/2+T2/2+T0/4];

switch (N)
case 0
    Ta = Tall(1);
    Tb = Tall(2);
    Tc = Tall(4);
case 1
    Ta = Tall(3);
    Tb = Tall(1);
    Tc = Tall(4);
case 2
    Ta = Tall(4);
    Tb = Tall(1);
    Tc = Tall(2);
case 3
    Ta = Tall(4);
    Tb = Tall(3);
    Tc = Tall(1);
case 4
    Ta = Tall(2);
    Tb = Tall(4);
    Tc = Tall(1);
case 5
    Ta = Tall(1);
    Tb = Tall(4);
    Tc = Tall(3);
otherwise
    Ta = 0;
    Tb = 0;
    Tc = 0;
            
end

end
